simulink model "Pendulo"  (R2024b)
settings: Solver=VariableStepAuto  StartTime=0.0  StopTime=20  RelTol=1e-3
InitFcn:
  | ip=0.0079;
  | mc=0.7031;
  | lp=0.3302;
  | mp=0.23;
  | fc= 0;
  | beq=4.3;
  | g=9.81;
  | bp=0.0024;
settings Model: Creator=Fernando  LastModifiedBy=Fernando

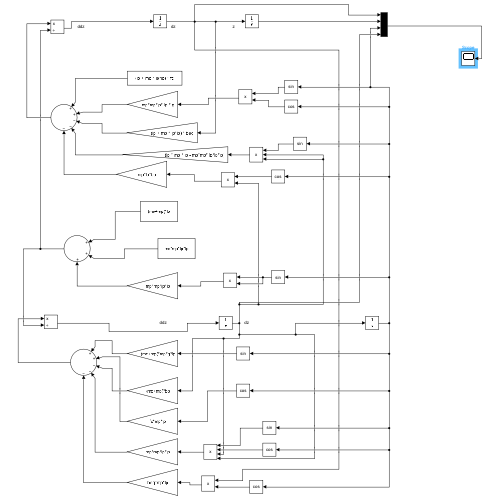
[thumbnail: Simulink's stored preview of the top-level diagram]
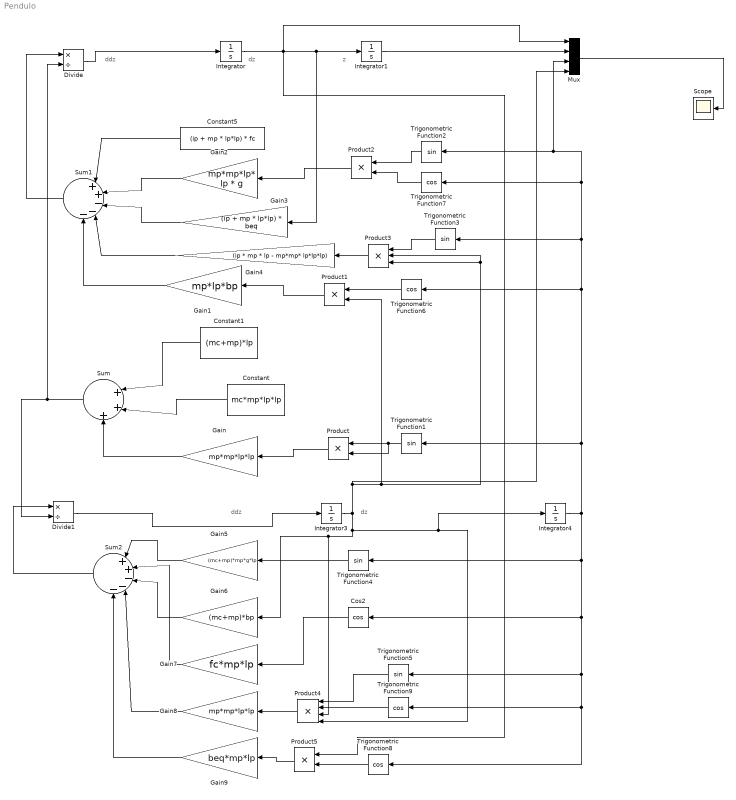
== system Pendulo ==
  note: dz
  note: ddz
  note: z
  note: dz
  note: ddz
  Constant : Constant  Value=mc*mp*lp*lp
  Constant1 : Constant  Value=(mc+mp)*lp
  Constant5 : Constant  Value=(ip + mp * lp*lp) * fc
  Cos2 : Trigonometry  Operator=cos
  Divide : Product  Inputs=*/
  Divide1 : Product  Inputs=*/
  Gain : Gain  Gain=mp*mp*lp*lp
  Gain1 : Gain  Gain=mp*lp*bp
  Gain2 : Gain  Gain=mp*mp*lp* lp * g
  Gain3 : Gain  Gain=(ip + mp * lp*lp) * beq
  Gain4 : Gain  Gain=(ip * mp * lp - mp*mp* lp*lp*lp)
  Gain5 : Gain  Gain=(mc+mp)*mp*g*lp
  Gain6 : Gain  Gain=(mc+mp)*bp
  Gain7 : Gain  Gain=fc*mp*lp
  Gain8 : Gain  Gain=mp*mp*lp*lp
  Gain9 : Gain  Gain=beq*mp*lp
  Integrator : Integrator
  Integrator1 : Integrator
  Integrator3 : Integrator
  Integrator4 : Integrator  InitialCondition=3.14/180
  Mux : Mux
  Product{,1..2,5} (4 alike) : Product
  Product3 : Product  Inputs=3
  Product4 : Product  Inputs=4
  Scope : Scope
  Sum : Sum  Inputs=|+++
  Sum1 : Sum  Inputs=|++---
  Sum2 : Sum  Inputs=|++---
  Trigonometric Function{1..5} (5 alike) : Trigonometry
  Trigonometric Function{6..9} (4 alike) : Trigonometry  Operator=cos
  wires:
  Constant1/1 -> Sum/1
  Constant/1 -> Sum/2
  Gain/1 -> Sum/3
  Product/1 -> Gain/1
  Trigonometric Function1/1 -> Product/2, Product/1
  Integrator/1 -> Integrator1/1, Gain3/1, Mux/1, Product5/1
  Integrator1/1 -> Mux/2
  Mux/1 -> Scope/1
  Product1/1 -> Gain1/1
  Constant5/1 -> Sum1/1
  Gain2/1 -> Sum1/2
  Gain3/1 -> Sum1/3
  Gain4/1 -> Sum1/4
  Gain1/1 -> Sum1/5
  Divide/1 -> Integrator/1
  Sum1/1 -> Divide/1
  Sum/1 -> Divide1/2, Divide/2
  Divide1/1 -> Integrator3/1
  Integrator3/1 -> Product4/3, Gain6/1, Product4/4, Integrator4/1, Product3/2, Product3/3, Product1/2, Mux/4
  Gain9/1 -> Sum2/5
  Gain8/1 -> Sum2/4
  Gain6/1 -> Sum2/3
  Gain7/1 -> Sum2/2
  Gain5/1 -> Sum2/1
  Sum2/1 -> Divide1/1
  Product2/1 -> Gain2/1
  Trigonometric Function2/1 -> Product2/1
  Trigonometric Function7/1 -> Product2/2
  Product3/1 -> Gain4/1
  Trigonometric Function3/1 -> Product3/1
  Trigonometric Function6/1 -> Product1/1
  Trigonometric Function4/1 -> Gain5/1
  Product4/1 -> Gain8/1
  Trigonometric Function5/1 -> Product4/1
  Trigonometric Function9/1 -> Product4/2
  Product5/1 -> Gain9/1
  Trigonometric Function8/1 -> Product5/2
  Integrator4/1 -> Trigonometric Function8/1, Trigonometric Function9/1, Trigonometric Function5/1, Cos2/1, Trigonometric Function4/1, Trigonometric Function6/1, Trigonometric Function7/1, Mux/3, Trigonometric Function2/1, Trigonometric Function3/1, Trigonometric Function1/1
  Cos2/1 -> Gain7/1
